simulink model "PIDdiscret_0001"  (Simulink 8.5)
settings: Solver=ode3  StartTime=0.0  StopTime=7  FixedStep=0.001  RelTol=1e-3
values from neighbouring files (symbols this model uses):
  K = (y_real(end) - y_real(1))/(input.signals.values(end) - 0)    [ctr.m]
  L = 1.5*(t1_28 - (t2_63/3))    [ctr.m]
  T = 1.5*(t2_63 - t1_28)    [ctr.m]
settings Model: Creator=guima  LastModifiedBy=guima
settings DataIOCC: SignalLoggingSaveFormat=Dataset
settings OptimizationCC: ExpressionDepthLimit=128
settings DebuggingCC: UnderspecifiedInitializationDetection=Simplified  MergeDetectMultiDrivingBlocksExec=error  FcnCallInpInsideContextMsg=EnableAllAsError  StateNameClashWarn=none
settings GRTTargetCC: CombineOutputUpdateFcns=on  GRTInterface=off

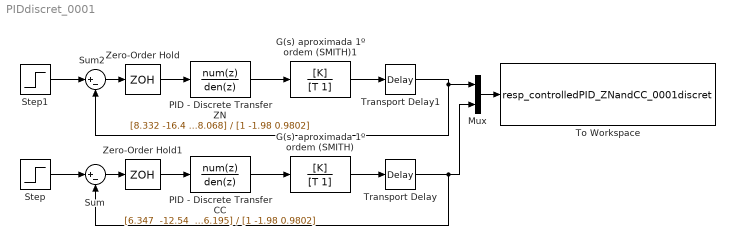
== system PIDdiscret_0001 ==
  G(s) aproximada 1º ordem (SMITH) : TransferFcn  Numerator=[K]  Denominator=[T 1]
  G(s) aproximada 1º ordem (SMITH)1 : TransferFcn  Numerator=[K]  Denominator=[T 1]
  Mux : Mux  Inputs=2
  PID - Discrete Transfer CC : DiscreteTransferFcn  Numerator="[6.347  -12.54  6.195]"  Denominator=[1 -1.98 0.9802]  SampleTime=0.001
  PID - Discrete Transfer ZN : DiscreteTransferFcn  Numerator=[8.332 -16.4 8.068]  Denominator=[1 -1.98 0.9802]  SampleTime=0.001
  Step : Step  Time=0  SampleTime=0
  Step1 : Step  Time=0  SampleTime=0
  Sum : Sum  Inputs=|+-
  Sum2 : Sum  Inputs=|+-
  To Workspace : ToWorkspace  VariableName=resp_controlledPID_ZNandCC_0001discret  SaveFormat=Structure With Time  SampleTime=-1
  Transport Delay : TransportDelay  DelayTime=L
  Transport Delay1 : TransportDelay  DelayTime=L
  Zero-Order Hold : ZeroOrderHold  SampleTime=0.001
  Zero-Order Hold1 : ZeroOrderHold  SampleTime=0.001
  wires:
  Step/1 -> Sum/1
  Sum/1 -> Zero-Order Hold1/1
  PID - Discrete Transfer CC/1 -> G(s) aproximada 1º ordem (SMITH)/1
  G(s) aproximada 1º ordem (SMITH)/1 -> Transport Delay/1
  Transport Delay/1 -> Mux/2, Sum/2
  Step1/1 -> Sum2/1
  G(s) aproximada 1º ordem (SMITH)1/1 -> Transport Delay1/1
  Transport Delay1/1 -> Mux/1, Sum2/2
  Mux/1 -> To Workspace/1
  Sum2/1 -> Zero-Order Hold/1
  PID - Discrete Transfer ZN/1 -> G(s) aproximada 1º ordem (SMITH)1/1
  Zero-Order Hold1/1 -> PID - Discrete Transfer CC/1
  Zero-Order Hold/1 -> PID - Discrete Transfer ZN/1
